simulink model "BEX6_USB_Torque_Control_HallSensor_BLDC_PMSM_2022b"  (R2022b)
settings: Solver=VariableStepAuto  StartTime=0.0  StopTime=inf  RelTol=1e-3
(part 1 of 2)
settings Model: Creator=SL_1  LastModifiedBy=SL_1
settings DebuggingCC: UnconnectedInputMsg=warning  UnconnectedOutputMsg=warning  UnconnectedLineMsg=warning
settings ModelReferenceCC: EnableRefExpFcnMdlSchedulingChecks=on
settings RTWCC: DLArmComputeVersion=19.05

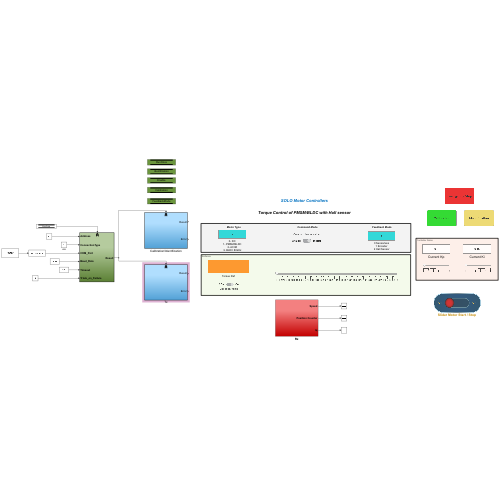
[thumbnail: Simulink's stored preview of the top-level diagram]
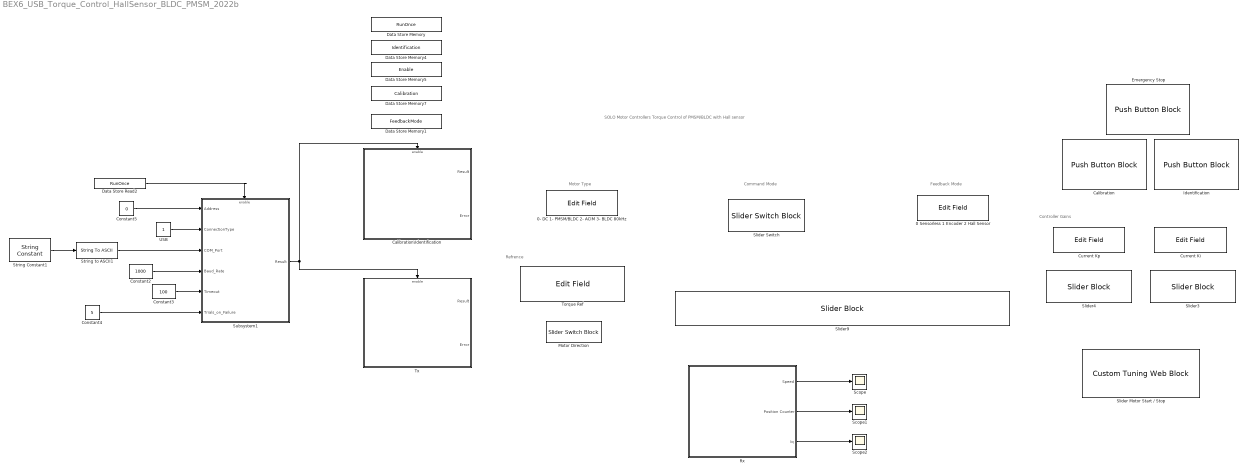
== system BEX6_USB_Torque_Control_HallSensor_BLDC_PMSM_2022b ==
  note: Command Mode
  note: Feedback Mode
  note: Refrence
  note: Controller Gains
  note: SOLO Motor Controllers
      |
      | Torque Control of PMSM/BLDC with Hall sensor
  note: Motor Type
  0 Sensorless 1 Encoder 2 Hall Sensor : EditField  LabelPosition=Hide  ShowInitialText=on  Alignment=Center
  "0- DC 1- PMSM/BLDC 2- ACIM 3- BLDC 80kHz " : EditField  LabelPosition=Hide  ShowInitialText=on  Alignment=Center
  Calibration : PushButtonBlock  ButtonText=Calibration  OffValue=0.000000
  Calibration\Identification : Subsystem
  Constant2 : Constant  Value=1000  OutDataTypeStr=uint32
  Constant3 : Constant  Value=100  OutDataTypeStr=double
  Constant4 : Constant  Value=5  OutDataTypeStr=int32
  Constant5 : Constant  Value=0  OutDataTypeStr=uint8
  Current Ki : EditField  LabelPosition=Hide  ShowInitialText=on  Alignment=Center
  Current Kp : EditField  LabelPosition=Hide  ShowInitialText=on  Alignment=Center
  Data Store Memory : DataStoreMemory  DataStoreName=RunOnce  ReadBeforeWriteMsg=warning  WriteAfterWriteMsg=warning  WriteAfterReadMsg=warning  InitialValue=1  ShowAdditionalParam=off  OutDataTypeStr=boolean
  Data Store Memory1 : DataStoreMemory  DataStoreName=FeedbackMode  ReadBeforeWriteMsg=warning  WriteAfterWriteMsg=warning  WriteAfterReadMsg=warning  ShowAdditionalParam=off
  Data Store Memory4 : DataStoreMemory  DataStoreName=Identification  ReadBeforeWriteMsg=warning  WriteAfterWriteMsg=warning  WriteAfterReadMsg=warning  ShowAdditionalParam=off
  Data Store Memory5 : DataStoreMemory  DataStoreName=Enable  ReadBeforeWriteMsg=warning  WriteAfterWriteMsg=warning  WriteAfterReadMsg=warning  ShowAdditionalParam=off
  Data Store Memory7 : DataStoreMemory  DataStoreName=Calibration  ReadBeforeWriteMsg=warning  WriteAfterWriteMsg=warning  WriteAfterReadMsg=warning  ShowAdditionalParam=off
  Data Store Read2 : DataStoreRead  DataStoreName=RunOnce  IndexOptions=Index vector (dialog)  Indices=1  OutputSizes=1
  Emergency Stop : PushButtonBlock  ButtonText=Emergency Stop  OnValue=0  OffValue=1.000000
  Identification : PushButtonBlock  ButtonText=Identification  OffValue=0.000000
  Motor Direction : SliderSwitchBlock  LabelPosition=Bottom
      settings: Values={{'CCw', 'Cw'}, [1 0]}
  Rx : Subsystem
  Scope : Scope
  Scope1 : Scope
  Scope2 : Scope
  Slider Motor Start / Stop : CustomTuningWebBlock  LabelPosition=Hide  ShowInitialText=on  Configuration="{\"type\":\"Switch\",\"settings\":{\"BindingType\":\"param\",\"backgroundColor\":[0,0,255,\"1\"],\"fixedAspectRatio\":\"on\",\"foregroundColor\":[234,234,234],\"showBackgroundColor\":false,\"variant\":\"slider\",\"version\":\"R2022b\"},\"components\":[{\"name\":\"CustomSwitchStateComponent\",\"settings\":{\"position\":[0,0,1,1],\"states\":[{\"HitRegion\":{\"position\":[0,0,0.5,1]},\"Image\":{\"position\":[0,0,1,1],\"size\":[1,1],\"src\":\"data:image/svg+xml;base64,PD94bWwgdmVyc2lvbj0iMS4wIiBlbmNvZGluZz0idXRmLTgiPz4NCjwhLS0gR2VuZXJhdG9yOiBBZG9iZSBJbGx1c3RyYXRvciAyNS4yLjEsIFNWRyBFeHBvcnQgUGx1Zy1JbiAuIFNWRyBWZXJzaW9uOiA2LjAwIEJ1aWxkIDApICAtLT4NCjxzdmcgdmVyc2lvbj0iMS4xIiB4bWxucz0iaHR0cDovL3d3dy53My5vcmcvMjAwMC9zdmciIHhtbG5zOnhsaW5rPSJodHRwOi8vd3d3LnczLm9yZy8xOTk5L3hsaW5rIiB4PSIwcHgiIHk9IjBweCINCgkgdmlld0JveD0iMCAwIDc2IDI5IiBzdHlsZT0iZW5hYmxlLWJhY2tncm91bmQ6bmV3 ...(+5404 chars)\",\"srcOrientation\":\"Right\"},\"Label\":{\"color\":[0.9294117647058824,0.6941176470588235,0.12549019607843137],\"icon\":{\"size\":[0,0],\"src\":[],\"srcOrientation\":\"Right\"},\"iconPlacement\":\"left\",\"opacity\":1,\"position\":[0.5,0.14],\"show\":true,\"text\":{\"content\":\"Off\",\"font\":\"Helvetica\",\"fontSize\":9}},\"Value\":0},{\"HitRegion\":{\"position\":[0,0.5,0.5,1]},\"Image\":{\"position\":[0,0,1,1],\"size\":[1,1],\"src\":\"data:image/svg+xml;base64,PD94bWwgdmVyc2lvbj0iMS4wIiBlbmNvZGluZz0idXRmLTgiPz4NCjwhLS0gR2VuZXJhdG9yOiBBZG9iZSBJbGx1c3RyYXRvciAyNS4yLjEsIFNWRyBFeHBvcnQgUGx1Zy1JbiAuIFNWRyBWZXJzaW9uOiA2LjAwIEJ1aWxkIDApICAtLT4NCjxzdmcgdmVyc2lvbj0iMS4xIiB4bWxucz0iaHR0cDovL3d3dy53My5vcmcvMjAwMC9zdmciIHhtbG5zOnhsaW5rPSJodHRwOi8vd3d3LnczLm9yZy8xOTk5L3hsaW5rIiB4PSIwcHgiIHk9IjBweCINCgkgdmlld0JveD0iMCAwIDc2IDI5IiBzdHlsZT0iZW5hYmxlLWJhY2tncm91bmQ6bmV3 ...(+5404 chars)\",\"srcOrientation\":\"Right\"},\"Label\":{\"color\":[0.9294117647058824,0.6941176470588235,0.12549019607843137],\"icon\":{\"size\":[0,0],\"src\":[],\"srcOrientation\":\"Right\"},\"iconPlacement\":\"left\",\"opacity\":1,\"position\":[0.5,0.86],\"show\":true,\"text\":{\"content\":\"On\",\"font\":\"Helvetica\",\"fontSize\":9}},\"Value\":1}]}},{\"name\":\"BackgroundImageComponent\",\"settings\":{\"image\":{\"size\":[0,0],\"src\":\"default\",\"srcOrientation\":[]},\"position\":[0,0,1,1],\"scaleMode\":\"0\"}},{\"name\":\"ForegroundImageComponent\",\"settings\":{\"image\":{\"size\":[0,0],\"src\":\"default\",\"srcOrientation\":[]},\"isForeground\":1,\"position\":[0,0,1,1],\"scaleMode\":\"0\"}}]}"
  Slider Switch : SliderSwitchBlock
      settings: Values={{'Analog', 'Digital'}, [0 1]}
  Slider3 : SliderBlock  LabelPosition=Hide  ScaleMax=5
  Slider4 : SliderBlock  LabelPosition=Hide  ScaleMax=5
  Slider9 : SliderBlock  LabelPosition=Hide  ScaleMax=3
  String Constant1 : StringConstant  String="\"COM5\""
  String to ASCII1 : StringToASCII  OutputVectorSize=5
  Subsystem1 : Subsystem
  Torque Ref : EditField  LabelPosition=Hide  ShowInitialText=on  Alignment=Center
  Tx : Subsystem
  USB : Constant  OutDataTypeStr=uint8
  wires:
  Rx/1(Speed) -> Scope/1
  Rx/2(Position Counter) -> Scope1/1
  Rx/3(Iq) -> Scope2/1
  Subsystem1/1(Result) -> Calibration\Identification/Enable, Tx/Enable
  Constant3/1 -> Subsystem1/5(Timeout)
  String to ASCII1/1 -> Subsystem1/3(COM_Port)
  Constant4/1 -> Subsystem1/6(Trials_on_Failure)
  Constant5/1 -> Subsystem1/1(Address)
  Constant2/1 -> Subsystem1/4(Baud_Rate)
  Data Store Read2/1 -> Subsystem1/Enable
  String Constant1/1 -> String to ASCII1/1
  USB/1 -> Subsystem1/2(ConnectionType)

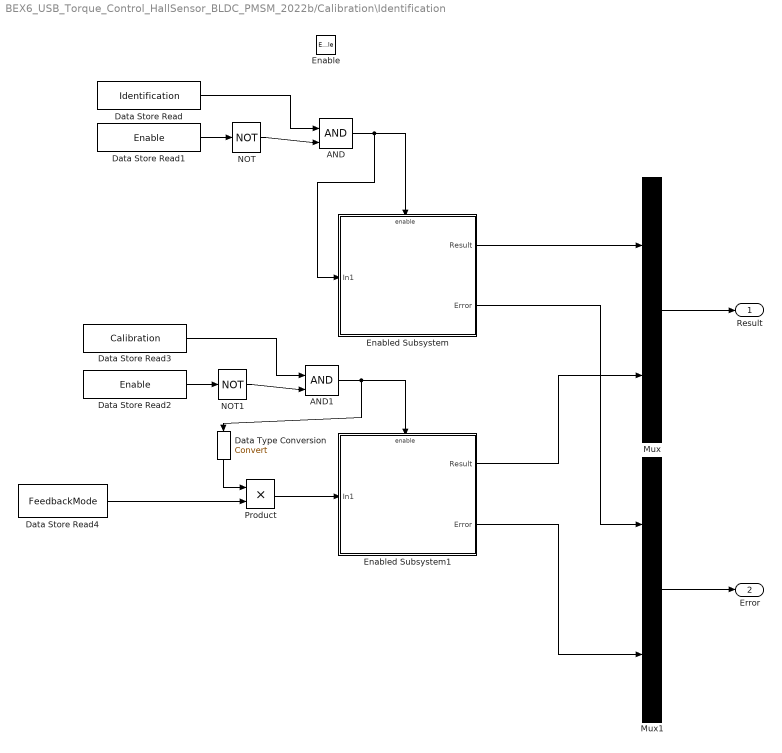
== system BEX6_USB_Torque_Control_HallSensor_BLDC_PMSM_2022b/Calibration\Identification ==
  Enable : EnablePort
  AND : Logic  IconShape=distinctive  AllPortsSameDT=off  OutDataTypeStr=boolean
  AND1 : Logic  IconShape=distinctive  AllPortsSameDT=off  OutDataTypeStr=boolean
  Data Store Read : DataStoreRead  DataStoreName=Identification  IndexOptions=Index vector (dialog)  Indices=1  OutputSizes=1
  Data Store Read1 : DataStoreRead  DataStoreName=Enable  IndexOptions=Index vector (dialog)  Indices=1  OutputSizes=1
  Data Store Read2 : DataStoreRead  DataStoreName=Enable  IndexOptions=Index vector (dialog)  Indices=1  OutputSizes=1
  Data Store Read3 : DataStoreRead  DataStoreName=Calibration  IndexOptions=Index vector (dialog)  Indices=1  OutputSizes=1
  Data Store Read4 : DataStoreRead  DataStoreName=FeedbackMode  IndexOptions=Index vector (dialog)  Indices=1  OutputSizes=1
  Data Type Conversion : DataTypeConversion  SaturateOnIntegerOverflow=off  RndMeth=Floor
  Enabled Subsystem : Subsystem  TreatAsAtomicUnit=on
  Enabled Subsystem1 : Subsystem  TreatAsAtomicUnit=on
  Mux : Mux  Inputs=2
  Mux1 : Mux  Inputs=2
  NOT : Logic  Operator=NOT  IconShape=distinctive  AllPortsSameDT=off  OutDataTypeStr=boolean
  NOT1 : Logic  Operator=NOT  IconShape=distinctive  AllPortsSameDT=off  OutDataTypeStr=boolean
  Product : Product
  Result : Outport
  Error : Outport  Port=2
  wires:
  Data Store Read1/1 -> NOT/1
  AND/1 -> Enabled Subsystem/1(In1), Enabled Subsystem/Enable
  NOT/1 -> AND/2
  Data Store Read/1 -> AND/1
  NOT1/1 -> AND1/2
  Data Store Read2/1 -> NOT1/1
  AND1/1 -> Data Type Conversion/1, Enabled Subsystem1/Enable
  Data Store Read3/1 -> AND1/1
  Enabled Subsystem1/2(Error) -> Mux1/2
  Enabled Subsystem1/1(Result) -> Mux/2
  Enabled Subsystem/1(Result) -> Mux/1
  Enabled Subsystem/2(Error) -> Mux1/1
  Mux1/1 -> Error/1
  Mux/1 -> Result/1
  Data Store Read4/1 -> Product/2
  Data Type Conversion/1 -> Product/1
  Product/1 -> Enabled Subsystem1/1(In1)

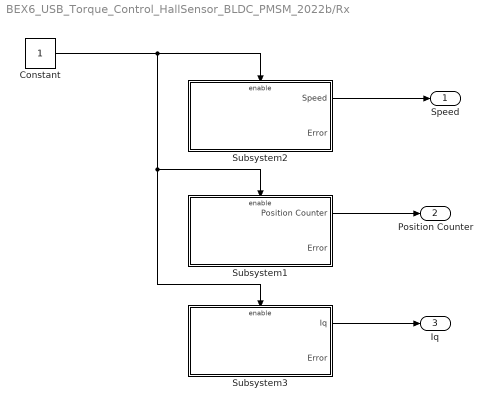
== system BEX6_USB_Torque_Control_HallSensor_BLDC_PMSM_2022b/Rx ==
  Constant : Constant  SampleTime=1e-3
  Subsystem1 : Subsystem
  Subsystem2 : Subsystem
  Subsystem3 : Subsystem
  Speed : Outport
  Position Counter : Outport  Port=2
  Iq : Outport  Port=3
  wires:
  Constant/1 -> Subsystem1/Enable, Subsystem3/Enable, Subsystem2/Enable
  Subsystem2/1(Speed) -> Speed/1
  Subsystem1/1(Position Counter) -> Position Counter/1
  Subsystem3/1(Iq) -> Iq/1

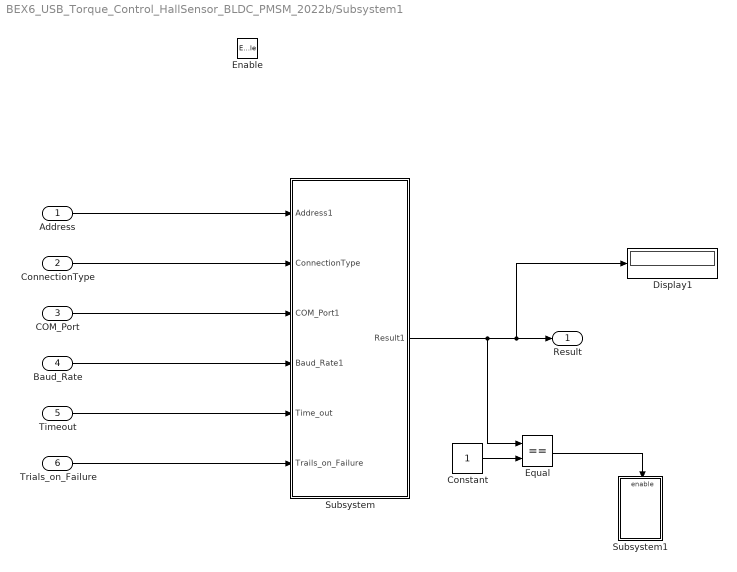
== system BEX6_USB_Torque_Control_HallSensor_BLDC_PMSM_2022b/Subsystem1 ==
  Address : Inport
  ConnectionType : Inport  Port=2
  COM_Port : Inport  Port=3
  Baud_Rate : Inport  Port=4
  Timeout : Inport  Port=5
  Trials_on_Failure : Inport  Port=6
  Enable : EnablePort
  Constant : Constant  OutDataTypeStr=Inherit: Inherit via back propagation
  Display1 : Display
  Equal : RelationalOperator  Operator===  OutDataTypeStr=boolean  RndMeth=Simplest  InputSameDT=off
  Subsystem : Subsystem
  Subsystem1 : Subsystem
  Result : Outport
  wires:
  Address/1 -> Subsystem/1(Address1)
  COM_Port/1 -> Subsystem/3(COM_Port1)
  Baud_Rate/1 -> Subsystem/4(Baud_Rate1)
  Timeout/1 -> Subsystem/5(Time_out)
  Trials_on_Failure/1 -> Subsystem/6(Trails_on_Failure)
  Equal/1 -> Subsystem1/Enable
  Subsystem/1(Result1) -> Display1/1, Result/1, Equal/1
  Constant/1 -> Equal/2
  ConnectionType/1 -> Subsystem/2(ConnectionType)

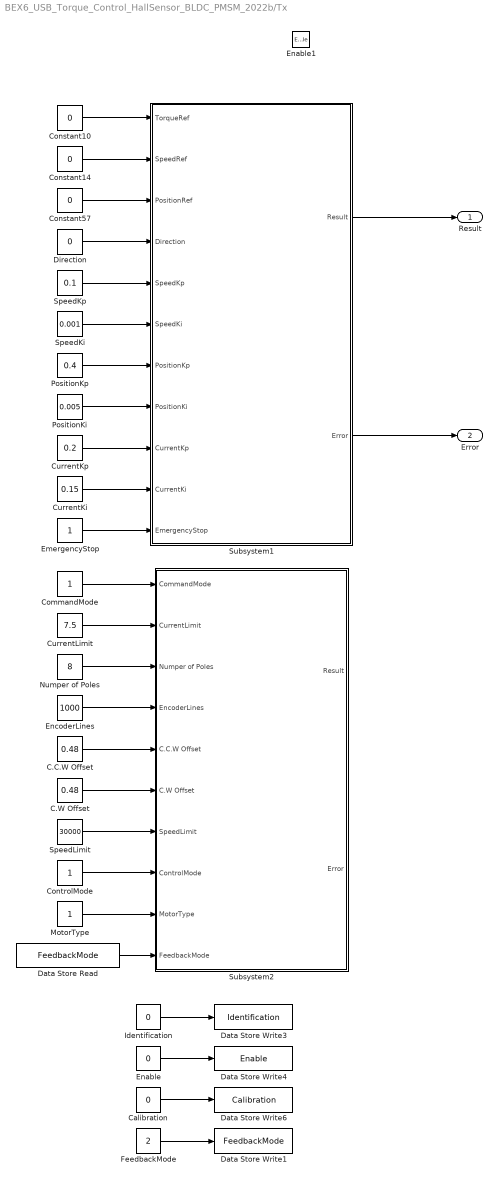
== system BEX6_USB_Torque_Control_HallSensor_BLDC_PMSM_2022b/Tx ==
  Enable1 : EnablePort
  C.C.W Offset : Constant  Value=0.48  OutDataTypeStr=Inherit: Inherit via back propagation
  C.W Offset : Constant  Value=0.48  OutDataTypeStr=Inherit: Inherit via back propagation
  Calibration : Constant  Value=0  OutDataTypeStr=Inherit: Inherit via back propagation
  CommandMode : Constant  OutDataTypeStr=Inherit: Inherit via back propagation
  Constant10 : Constant  Value=0  OutDataTypeStr=Inherit: Inherit via back propagation
  Constant14 : Constant  Value=0  OutDataTypeStr=Inherit: Inherit via back propagation
  Constant57 : Constant  Value=0  OutDataTypeStr=int32
  ControlMode : Constant  OutDataTypeStr=Inherit: Inherit via back propagation
  CurrentKi : Constant  Value=0.15  OutDataTypeStr=Inherit: Inherit via back propagation
  CurrentKp : Constant  Value=0.2  OutDataTypeStr=Inherit: Inherit via back propagation
  CurrentLimit : Constant  Value=7.5  OutDataTypeStr=Inherit: Inherit via back propagation
  Data Store Read : DataStoreRead  DataStoreName=FeedbackMode  IndexOptions=Index vector (dialog)  Indices=1  OutputSizes=1
  Data Store Write1 : DataStoreWrite  DataStoreName=FeedbackMode  IndexOptions=Index vector (dialog)  Indices=1  OutputSizes=1
  Data Store Write3 : DataStoreWrite  DataStoreName=Identification  IndexOptions=Index vector (dialog)  Indices=1  OutputSizes=1
  Data Store Write4 : DataStoreWrite  DataStoreName=Enable  IndexOptions=Index vector (dialog)  Indices=1  OutputSizes=1
  Data Store Write6 : DataStoreWrite  DataStoreName=Calibration  IndexOptions=Index vector (dialog)  Indices=1  OutputSizes=1
  Direction : Constant  Value=0  OutDataTypeStr=Inherit: Inherit via back propagation
  EmergencyStop : Constant  OutDataTypeStr=boolean
  Enable : Constant  Value=0  OutDataTypeStr=Inherit: Inherit via back propagation
  EncoderLines : Constant  Value=1000  OutDataTypeStr=Inherit: Inherit via back propagation
  FeedbackMode : Constant  Value=2  OutDataTypeStr=Inherit: Inherit via back propagation
  Identification : Constant  Value=0  OutDataTypeStr=Inherit: Inherit via back propagation
  MotorType : Constant  OutDataTypeStr=Inherit: Inherit via back propagation
  Numper of Poles : Constant  Value=8  OutDataTypeStr=Inherit: Inherit via back propagation
  PositionKi : Constant  Value=0.005  OutDataTypeStr=Inherit: Inherit via back propagation
  PositionKp : Constant  Value=0.4  OutDataTypeStr=Inherit: Inherit via back propagation
  SpeedKi : Constant  Value=0.001  OutDataTypeStr=Inherit: Inherit via back propagation
  SpeedKp : Constant  Value=0.1  OutDataTypeStr=Inherit: Inherit via back propagation
  SpeedLimit : Constant  Value=30000  OutDataTypeStr=Inherit: Inherit via back propagation
  Subsystem1 : Subsystem
  Subsystem2 : Subsystem
  Result : Outport
  Error : Outport  Port=2
  wires:
  Direction/1 -> Subsystem1/4(Direction)
  Constant10/1 -> Subsystem1/1(TorqueRef)
  Constant14/1 -> Subsystem1/2(SpeedRef)
  Constant57/1 -> Subsystem1/3(PositionRef)
  CurrentKi/1 -> Subsystem1/10(CurrentKi)
  CurrentKp/1 -> Subsystem1/9(CurrentKp)
  PositionKi/1 -> Subsystem1/8(PositionKi)
  PositionKp/1 -> Subsystem1/7(PositionKp)
  SpeedKi/1 -> Subsystem1/6(SpeedKi)
  SpeedKp/1 -> Subsystem1/5(SpeedKp)
  Identification/1 -> Data Store Write3/1
  Enable/1 -> Data Store Write4/1
  EmergencyStop/1 -> Subsystem1/11(EmergencyStop)
  Subsystem1/1(Result) -> Result/1
  Subsystem1/2(Error) -> Error/1
  C.C.W Offset/1 -> Subsystem2/5(C.C.W Offset)
  Numper of Poles/1 -> Subsystem2/3(Numper of Poles)
  SpeedLimit/1 -> Subsystem2/7(SpeedLimit)
  C.W Offset/1 -> Subsystem2/6(C.W Offset)
  CommandMode/1 -> Subsystem2/1(CommandMode)
  EncoderLines/1 -> Subsystem2/4(EncoderLines)
  CurrentLimit/1 -> Subsystem2/2(CurrentLimit)
  MotorType/1 -> Subsystem2/9(MotorType)
  FeedbackMode/1 -> Data Store Write1/1
  Data Store Read/1 -> Subsystem2/10(FeedbackMode)
  ControlMode/1 -> Subsystem2/8(ControlMode)
  Calibration/1 -> Data Store Write6/1

== system BEX6_USB_Torque_Control_HallSensor_BLDC_PMSM_2022b/Calibration\Identification/Enabled Subsystem ==
  In1 : Inport
  Enable : EnablePort
  Constant21 : Constant  Value=0  OutDataTypeStr=uint8
  MotorParameterIdentification : Subsystem
  Result : Outport
  Error : Outport  Port=2
  wires:
  In1/1 -> MotorParameterIdentification/2(Value)
  Constant21/1 -> MotorParameterIdentification/1(Address)
  MotorParameterIdentification/2(Error) -> Error/1
  MotorParameterIdentification/1(Result) -> Result/1

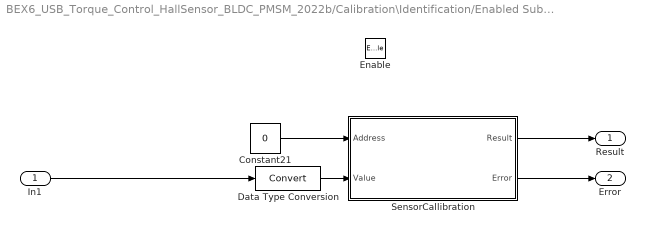
== system BEX6_USB_Torque_Control_HallSensor_BLDC_PMSM_2022b/Calibration\Identification/Enabled Subsystem1 ==
  In1 : Inport
  Enable : EnablePort
  Constant21 : Constant  Value=0  OutDataTypeStr=uint8
  Data Type Conversion : DataTypeConversion  SaturateOnIntegerOverflow=off  RndMeth=Floor
  SensorCallibration : Subsystem
  Result : Outport
  Error : Outport  Port=2
  wires:
  Constant21/1 -> SensorCallibration/1(Address)
  In1/1 -> Data Type Conversion/1
  Data Type Conversion/1 -> SensorCallibration/2(Value)
  SensorCallibration/2(Error) -> Error/1
  SensorCallibration/1(Result) -> Result/1

== system BEX6_USB_Torque_Control_HallSensor_BLDC_PMSM_2022b/Rx/Subsystem1 ==
  Enable : EnablePort
  Constant120 : Constant  Value=0  OutDataTypeStr=uint8
  GetPositionCountsFeedback : Subsystem
  Position Counter : Outport
  Error : Outport  Port=2
  wires:
  Constant120/1 -> GetPositionCountsFeedback/1(Address)
  GetPositionCountsFeedback/1(Result) -> Position Counter/1
  GetPositionCountsFeedback/2(Error) -> Error/1

== system BEX6_USB_Torque_Control_HallSensor_BLDC_PMSM_2022b/Rx/Subsystem2 ==
  Enable : EnablePort
  Constant120 : Constant  Value=0  OutDataTypeStr=uint8
  GetSpeedFeedback : Subsystem
  Speed : Outport
  Error : Outport  Port=2
  wires:
  GetSpeedFeedback/1(Result) -> Speed/1
  Constant120/1 -> GetSpeedFeedback/1(Address)
  GetSpeedFeedback/2(Error) -> Error/1

== system BEX6_USB_Torque_Control_HallSensor_BLDC_PMSM_2022b/Rx/Subsystem3 ==
  Enable : EnablePort
  Constant120 : Constant  Value=0  OutDataTypeStr=uint8
  GetQuadratureCurrentIqFeedback : Subsystem
  Iq : Outport
  Error : Outport  Port=2
  wires:
  GetQuadratureCurrentIqFeedback/2(Error) -> Error/1
  GetQuadratureCurrentIqFeedback/1(Result) -> Iq/1
  Constant120/1 -> GetQuadratureCurrentIqFeedback/1(Address)

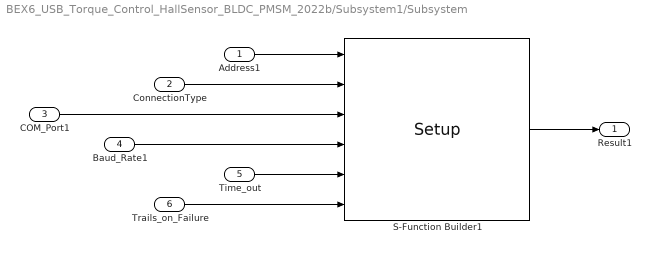
== system BEX6_USB_Torque_Control_HallSensor_BLDC_PMSM_2022b/Subsystem1/Subsystem ==
  Address1 : Inport
  ConnectionType : Inport  Port=2
  COM_Port1 : Inport  Port=3
  Baud_Rate1 : Inport  Port=4
  Time_out : Inport  Port=5
  Trails_on_Failure : Inport  Port=6
  S-Function Builder1 : S-Function  Priority=1  FunctionName=Setup  SFunctionModules=Setup_wrapper  SFunctionDeploymentMode=off  EnableBusSupport=off  mask(S-Function Builder){}
      mask help: Simulink:masks:SFunctionBuilder_MD
      mask init:
      | val = [[.9  0.75 0.75 1 1 .9 .9 1]',[1 1 0.75 0.75 .9 .9 1 .9]'];try , sys = get_param(gcb,'SfunBuilderFcnName');if isempty(sys), sys = get_param(gcb,'FunctionName'); end,catch, sys = get_param(gcb,'FunctionName'); end
      settings: CopyFcn=set_param(gcbh,'LinkStatus','none')  OpenFcn=sfunctionwizard(gcbh)
      mask Display:
      | plot(val(:,1),val(:,2))
      | disp(sys)
      | port_label('input',1,'Address')
      | port_label('input',2,'ConnectionType')
      | port_label('input',3,'COM_Port')
      | port_label('input',4,'Baud_Rate')
      | port_label('input',5,'Timeout')
      | port_label('input',6,'Trials_on_Failure')
      | port_label('output',1,'Result')
  Result1 : Outport
  wires:
  ConnectionType/1 -> S-Function Builder1/2
  Address1/1 -> S-Function Builder1/1
  S-Function Builder1/1 -> Result1/1
  Trails_on_Failure/1 -> S-Function Builder1/6
  COM_Port1/1 -> S-Function Builder1/3
  Time_out/1 -> S-Function Builder1/5
  Baud_Rate1/1 -> S-Function Builder1/4

== system BEX6_USB_Torque_Control_HallSensor_BLDC_PMSM_2022b/Subsystem1/Subsystem1 ==
  Enable : EnablePort
  Constant1 : Constant  Value=0  OutDataTypeStr=Inherit: Inherit via back propagation
  Data Store Write : DataStoreWrite  DataStoreName=RunOnce  IndexOptions=Index vector (dialog)  Indices=1  OutputSizes=1
  wires:
  Constant1/1 -> Data Store Write/1

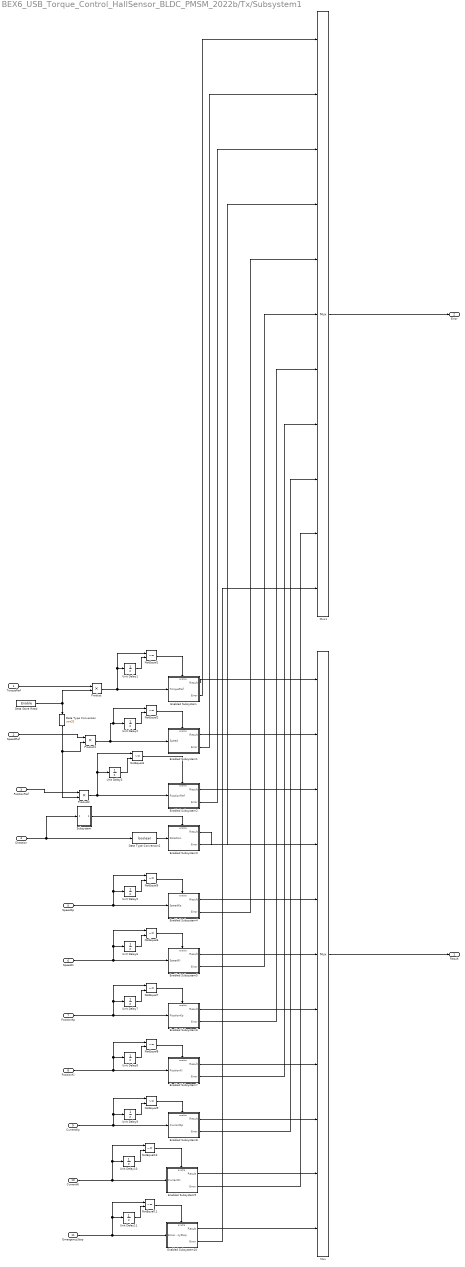
== system BEX6_USB_Torque_Control_HallSensor_BLDC_PMSM_2022b/Tx/Subsystem1 ==
  TorqueRef : Inport
  SpeedRef : Inport  Port=2
  PositionRef : Inport  Port=3
  Direction : Inport  Port=4
  SpeedKp : Inport  Port=5
  SpeedKi : Inport  Port=6
  PositionKp : Inport  Port=7
  PositionKi : Inport  Port=8
  CurrentKp : Inport  Port=9
  CurrentKi : Inport  Port=10
  EmergencyStop : Inport  Port=11
  Data Store Read : DataStoreRead  DataStoreName=Enable  IndexOptions=Index vector (dialog)  Indices=1  OutputSizes=1
  Data Type Conversion : DataTypeConversion  OutDataTypeStr=uint32  SaturateOnIntegerOverflow=off  RndMeth=Floor
  Data Type Conversion2 : DataTypeConversion  OutDataTypeStr=boolean  SaturateOnIntegerOverflow=off  RndMeth=Floor
  Enabled Subsystem : Subsystem  TreatAsAtomicUnit=on
  Enabled Subsystem1 : Subsystem  TreatAsAtomicUnit=on
  Enabled Subsystem10 : Subsystem  TreatAsAtomicUnit=on
  Enabled Subsystem2 : Subsystem  TreatAsAtomicUnit=on
  Enabled Subsystem3 : Subsystem  TreatAsAtomicUnit=on
  Enabled Subsystem4 : Subsystem  TreatAsAtomicUnit=on
  Enabled Subsystem5 : Subsystem  TreatAsAtomicUnit=on
  Enabled Subsystem6 : Subsystem  TreatAsAtomicUnit=on
  Enabled Subsystem7 : Subsystem  TreatAsAtomicUnit=on
  Enabled Subsystem8 : Subsystem  TreatAsAtomicUnit=on
  Enabled Subsystem9 : Subsystem  TreatAsAtomicUnit=on
  Mux : Mux  Inputs=11
  Mux1 : Mux  Inputs=11
  NotEqual{1..3,5..11} (10 alike) : RelationalOperator  Operator=~=  OutDataTypeStr=boolean  RndMeth=Simplest  InputSameDT=off
  Product : Product
  Product1 : Product  OutDataTypeStr=Inherit: Inherit via back propagation
  Product2 : Product  OutDataTypeStr=Inherit: Inherit via back propagation
  Subsystem : Subsystem
  Unit Delay{1..3,5..11} (10 alike) : UnitDelay  InitialCondition=2.1651  SampleTime=-1  HasFrameUpgradeWarning=on
  Result : Outport
  Error : Outport  Port=2
  wires:
  TorqueRef/1 -> Product/1
  Unit Delay1/1 -> NotEqual1/2
  NotEqual1/1 -> Enabled Subsystem/Enable
  Data Store Read/1 -> Product/2, Data Type Conversion/1
  Product/1 -> Enabled Subsystem/1(TorqueRef), NotEqual1/1, Unit Delay1/1
  NotEqual2/1 -> Enabled Subsystem1/Enable
  Unit Delay2/1 -> NotEqual2/2
  SpeedRef/1 -> Product1/1
  Product1/1 -> NotEqual2/1, Unit Delay2/1, Enabled Subsystem1/1(Speed)
  PositionRef/1 -> Product2/1
  Unit Delay3/1 -> NotEqual3/2
  NotEqual3/1 -> Enabled Subsystem2/Enable
  Direction/1 -> Data Type Conversion2/1, Subsystem/1(In1)
  NotEqual5/1 -> Enabled Subsystem4/Enable
  Unit Delay5/1 -> NotEqual5/2
  SpeedKp/1 -> Unit Delay5/1, NotEqual5/1, Enabled Subsystem4/1(SpeedKp)
  SpeedKi/1 -> NotEqual6/1, Unit Delay6/1, Enabled Subsystem5/1(SpeedKi)
  Unit Delay6/1 -> NotEqual6/2
  NotEqual6/1 -> Enabled Subsystem5/Enable
  NotEqual7/1 -> Enabled Subsystem6/Enable
  Unit Delay7/1 -> NotEqual7/2
  PositionKp/1 -> Unit Delay7/1, NotEqual7/1, Enabled Subsystem6/1(PositionKp)
  PositionKi/1 -> NotEqual8/1, Unit Delay8/1, Enabled Subsystem7/1(PositionKi)
  Unit Delay8/1 -> NotEqual8/2
  NotEqual8/1 -> Enabled Subsystem7/Enable
  NotEqual9/1 -> Enabled Subsystem8/Enable
  Unit Delay9/1 -> NotEqual9/2
  CurrentKp/1 -> Unit Delay9/1, NotEqual9/1, Enabled Subsystem8/1(CurrentKp)
  CurrentKi/1 -> NotEqual10/1, Unit Delay10/1, Enabled Subsystem9/1(CurrentKi)
  Unit Delay10/1 -> NotEqual10/2
  NotEqual10/1 -> Enabled Subsystem9/Enable
  NotEqual11/1 -> Enabled Subsystem10/Enable
  Unit Delay11/1 -> NotEqual11/2
  EmergencyStop/1 -> Unit Delay11/1, NotEqual11/1, Enabled Subsystem10/1(EmergencyStop)
  Product2/1 -> NotEqual3/1, Unit Delay3/1, Enabled Subsystem2/1(PositionRef)
  Data Type Conversion2/1 -> Enabled Subsystem3/1(Direction)
  Enabled Subsystem/1(Result) -> Mux/1
  Enabled Subsystem10/1(Result) -> Mux/11
  Enabled Subsystem9/1(Result) -> Mux/10
  Enabled Subsystem8/1(Result) -> Mux/9
  Enabled Subsystem7/1(Result) -> Mux/8
  Enabled Subsystem6/1(Result) -> Mux/7
  Enabled Subsystem5/1(Result) -> Mux/6
  Enabled Subsystem4/1(Result) -> Mux/5
  Enabled Subsystem3/1(Result) -> Mux/4
  Enabled Subsystem2/1(Result) -> Mux/3
  Enabled Subsystem1/1(Result) -> Mux/2
  Mux/1 -> Result/1
  Enabled Subsystem/2(Error) -> Mux1/1
  Enabled Subsystem1/2(Error) -> Mux1/2
  Enabled Subsystem2/2(Error) -> Mux1/3
  Enabled Subsystem3/2(Error) -> Mux1/4
  Enabled Subsystem4/2(Error) -> Mux1/5
  Enabled Subsystem5/2(Error) -> Mux1/6
  Enabled Subsystem6/2(Error) -> Mux1/7
  Enabled Subsystem7/2(Error) -> Mux1/8
  Enabled Subsystem8/2(Error) -> Mux1/9
  Enabled Subsystem9/2(Error) -> Mux1/10
  Enabled Subsystem10/2(Error) -> Mux1/11
  Mux1/1 -> Error/1
  Data Type Conversion/1 -> Product2/2, Product1/2
  Subsystem/1(Out1) -> Enabled Subsystem3/Enable

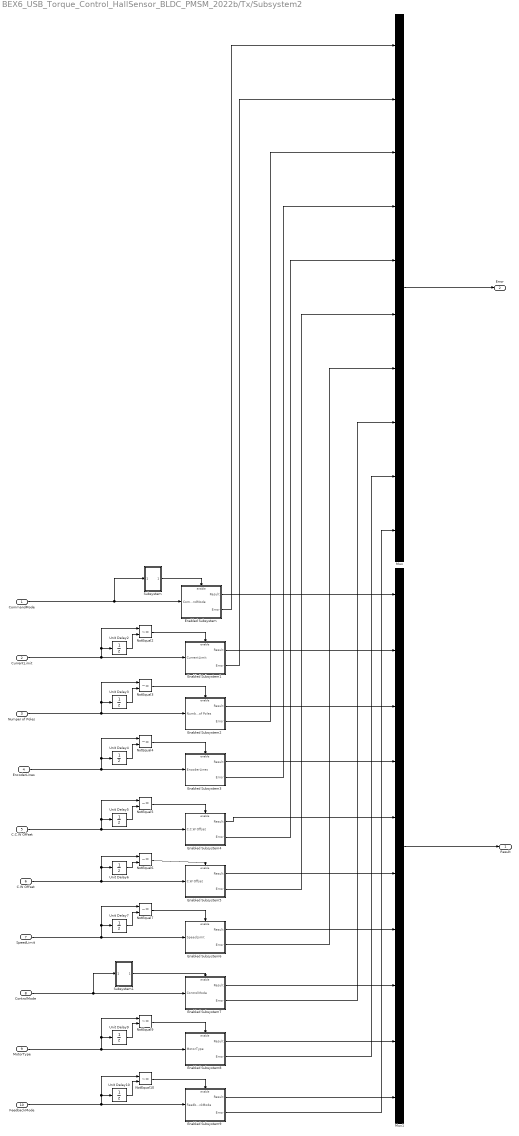
== system BEX6_USB_Torque_Control_HallSensor_BLDC_PMSM_2022b/Tx/Subsystem2 ==
  CommandMode : Inport
  CurrentLimit : Inport  Port=2
  Numper of Poles : Inport  Port=3
  EncoderLines : Inport  Port=4
  C.C.W Offset : Inport  Port=5
  C.W Offset : Inport  Port=6
  SpeedLimit : Inport  Port=7
  ControlMode : Inport  Port=8
  MotorType : Inport  Port=9
  FeedbackMode : Inport  Port=10
  Enabled Subsystem : Subsystem  TreatAsAtomicUnit=on
  Enabled Subsystem1 : Subsystem  TreatAsAtomicUnit=on
  Enabled Subsystem2 : Subsystem  TreatAsAtomicUnit=on
  Enabled Subsystem3 : Subsystem  TreatAsAtomicUnit=on
  Enabled Subsystem4 : Subsystem  TreatAsAtomicUnit=on
  Enabled Subsystem5 : Subsystem  TreatAsAtomicUnit=on
  Enabled Subsystem6 : Subsystem  TreatAsAtomicUnit=on
  Enabled Subsystem7 : Subsystem  TreatAsAtomicUnit=on
  Enabled Subsystem8 : Subsystem  TreatAsAtomicUnit=on
  Enabled Subsystem9 : Subsystem  TreatAsAtomicUnit=on
  Mux : Mux  Inputs=10
  Mux1 : Mux  Inputs=10
  NotEqual{2..7,9..10} (8 alike) : RelationalOperator  Operator=~=  OutDataTypeStr=boolean  RndMeth=Simplest  InputSameDT=off
  Subsystem : Subsystem
  Subsystem1 : Subsystem
  Unit Delay{2..7,9..10} (8 alike) : UnitDelay  InitialCondition=2.1651  SampleTime=-1  HasFrameUpgradeWarning=on
  Result : Outport
  Error : Outport  Port=2
  wires:
  NotEqual2/1 -> Enabled Subsystem1/Enable
  CurrentLimit/1 -> NotEqual2/1, Unit Delay2/1, Enabled Subsystem1/1(CurrentLimit)
  Unit Delay2/1 -> NotEqual2/2
  Unit Delay3/1 -> NotEqual3/2
  Numper of Poles/1 -> Enabled Subsystem2/1(Number of Poles), Unit Delay3/1, NotEqual3/1
  NotEqual3/1 -> Enabled Subsystem2/Enable
  NotEqual4/1 -> Enabled Subsystem3/Enable
  EncoderLines/1 -> NotEqual4/1, Unit Delay4/1, Enabled Subsystem3/1(EncoderLines)
  Unit Delay4/1 -> NotEqual4/2
  Unit Delay5/1 -> NotEqual5/2
  C.C.W Offset/1 -> Enabled Subsystem4/1(C.C.W Offset), Unit Delay5/1, NotEqual5/1
  NotEqual5/1 -> Enabled Subsystem4/Enable
  NotEqual6/1 -> Enabled Subsystem5/Enable
  C.W Offset/1 -> NotEqual6/1, Unit Delay6/1, Enabled Subsystem5/1(C.W Offset)
  Unit Delay6/1 -> NotEqual6/2
  Unit Delay7/1 -> NotEqual7/2
  SpeedLimit/1 -> Enabled Subsystem6/1(SpeedLimit), Unit Delay7/1, NotEqual7/1
  NotEqual7/1 -> Enabled Subsystem6/Enable
  ControlMode/1 -> Subsystem1/1(In1), Enabled Subsystem7/1(ControlMode)
  Unit Delay9/1 -> NotEqual9/2
  MotorType/1 -> Unit Delay9/1, NotEqual9/1, Enabled Subsystem8/1(MotorType)
  NotEqual9/1 -> Enabled Subsystem8/Enable
  NotEqual10/1 -> Enabled Subsystem9/Enable
  FeedbackMode/1 -> NotEqual10/1, Unit Delay10/1, Enabled Subsystem9/1(FeedbackMode)
  Unit Delay10/1 -> NotEqual10/2
  CommandMode/1 -> Subsystem/1(In1), Enabled Subsystem/1(CommandMode)
  Enabled Subsystem9/2(Error) -> Mux/10
  Enabled Subsystem8/2(Error) -> Mux/9
  Enabled Subsystem7/2(Error) -> Mux/8
  Enabled Subsystem6/2(Error) -> Mux/7
  Enabled Subsystem5/2(Error) -> Mux/6
  Enabled Subsystem4/2(Error) -> Mux/5
  Enabled Subsystem3/2(Error) -> Mux/4
  Enabled Subsystem2/2(Error) -> Mux/3
  Enabled Subsystem1/2(Error) -> Mux/2
  Enabled Subsystem/2(Error) -> Mux/1
  Enabled Subsystem/1(Result) -> Mux1/1
  Enabled Subsystem1/1(Result) -> Mux1/2
  Enabled Subsystem2/1(Result) -> Mux1/3
  Enabled Subsystem3/1(Result) -> Mux1/4
  Enabled Subsystem5/1(Result) -> Mux1/6
  Enabled Subsystem7/1(Result) -> Mux1/8
  Enabled Subsystem6/1(Result) -> Mux1/7
  Enabled Subsystem8/1(Result) -> Mux1/9
  Enabled Subsystem9/1(Result) -> Mux1/10
  Enabled Subsystem4/1(Result) -> Mux1/5
  Mux1/1 -> Result/1
  Mux/1 -> Error/1
  Subsystem/1(Out2) -> Enabled Subsystem/Enable
  Subsystem1/1(Out1) -> Enabled Subsystem7/Enable

== system BEX6_USB_Torque_Control_HallSensor_BLDC_PMSM_2022b/Calibration\Identification/Enabled Subsystem/MotorParameterIdentification ==
  Address : Inport
  Value : Inport  Port=2
  Display20 : Display
      settings: Format=decimal (Stored Integer)
  Display21 : Display
      settings: Format=decimal (Stored Integer)
  S-Function Builder10 : S-Function  Priority=2  FunctionName=MotorParametersIdentification  SFunctionModules=MotorParametersIdentification_wrapper  SFunctionDeploymentMode=off  EnableBusSupport=off  mask(S-Function Builder){}
      mask help: Simulink:masks:SFunctionBuilder_MD
      mask init: same as BEX6_USB_Torque_Control_HallSensor_BLDC_PMSM_2022b/Subsystem1/Subsystem/S-Function Builder1
      settings: CopyFcn=set_param(gcbh,'LinkStatus','none')  OpenFcn=sfunctionwizard(gcbh)
      mask Display:
      | plot(val(:,1),val(:,2))
      | disp(sys)
      | port_label('input',1,'Address')
      | port_label('input',2,'Value')
      | port_label('output',1,'Result')
      | port_label('output',2,'Error')
  Result : Outport
  Error : Outport  Port=2
  wires:
  S-Function Builder10/2 -> Error/1, Display21/1
  S-Function Builder10/1 -> Result/1, Display20/1
  Value/1 -> S-Function Builder10/2
  Address/1 -> S-Function Builder10/1

== system BEX6_USB_Torque_Control_HallSensor_BLDC_PMSM_2022b/Calibration\Identification/Enabled Subsystem1/SensorCallibration ==
  Address : Inport
  Value : Inport  Port=2
  S-Function Builder41 : S-Function  Priority=2  FunctionName=SensorCalibration  SFunctionModules=SensorCalibration_wrapper  SFunctionDeploymentMode=off  EnableBusSupport=off  mask(S-Function Builder){}
      mask help: Simulink:masks:SFunctionBuilder_MD
      mask init: same as BEX6_USB_Torque_Control_HallSensor_BLDC_PMSM_2022b/Subsystem1/Subsystem/S-Function Builder1
      settings: CopyFcn=set_param(gcbh,'LinkStatus','none')  OpenFcn=sfunctionwizard(gcbh)
      mask Display:
      | plot(val(:,1),val(:,2))
      | disp(sys)
      | port_label('input',1,'Address')
      | port_label('input',2,'Value')
      | port_label('output',1,'Result')
      | port_label('output',2,'Error')
  Result : Outport
  Error : Outport  Port=2
  wires:
  Value/1 -> S-Function Builder41/2
  S-Function Builder41/1 -> Result/1
  Address/1 -> S-Function Builder41/1
  S-Function Builder41/2 -> Error/1

== system BEX6_USB_Torque_Control_HallSensor_BLDC_PMSM_2022b/Rx/Subsystem1/GetPositionCountsFeedback ==
  Address : Inport
  S-Function Builder73 : S-Function  Priority=3  FunctionName=GetPositionCountsFeedback  SFunctionModules=GetPositionCountsFeedback_wrapper  SFunctionDeploymentMode=off  EnableBusSupport=off  mask(S-Function Builder){}
      mask help: Simulink:masks:SFunctionBuilder_MD
      mask init: same as BEX6_USB_Torque_Control_HallSensor_BLDC_PMSM_2022b/Subsystem1/Subsystem/S-Function Builder1
      settings: CopyFcn=set_param(gcbh,'LinkStatus','none')  OpenFcn=sfunctionwizard(gcbh)
      mask Display: plot(val(:,1),val(:,2)),disp(sys),port_label('input',1,'Address'),port_label('output',1,'Result'),port_label('output',2,'Error')
  Result : Outport
  Error : Outport  Port=2
  wires:
  Address/1 -> S-Function Builder73/1
  S-Function Builder73/2 -> Error/1
  S-Function Builder73/1 -> Result/1

== system BEX6_USB_Torque_Control_HallSensor_BLDC_PMSM_2022b/Rx/Subsystem2/GetSpeedFeedback ==
  Address : Inport
  S-Function Builder66 : S-Function  Priority=3  FunctionName=GetSpeedFeedback  SFunctionModules=GetSpeedFeedback_wrapper  SFunctionDeploymentMode=off  EnableBusSupport=off  mask(S-Function Builder){}
      mask help: Simulink:masks:SFunctionBuilder_MD
      mask init: same as BEX6_USB_Torque_Control_HallSensor_BLDC_PMSM_2022b/Subsystem1/Subsystem/S-Function Builder1
      settings: CopyFcn=set_param(gcbh,'LinkStatus','none')  OpenFcn=sfunctionwizard(gcbh)
      mask Display: plot(val(:,1),val(:,2)),disp(sys),port_label('input',1,'Address'),port_label('output',1,'Result'),port_label('output',2,'Error')
  Result : Outport
  Error : Outport  Port=2
  wires:
  Address/1 -> S-Function Builder66/1
  S-Function Builder66/1 -> Result/1
  S-Function Builder66/2 -> Error/1

== system BEX6_USB_Torque_Control_HallSensor_BLDC_PMSM_2022b/Rx/Subsystem3/GetQuadratureCurrentIqFeedback ==
  Address : Inport
  S-Function Builder57 : S-Function  Priority=3  FunctionName=GetQuadratureCurrentIqFeedback  SFunctionModules=GetQuadratureCurrentIqFeedback_wrapper  SFunctionDeploymentMode=off  EnableBusSupport=off  mask(S-Function Builder){}
      mask help: Simulink:masks:SFunctionBuilder_MD
      mask init: same as BEX6_USB_Torque_Control_HallSensor_BLDC_PMSM_2022b/Subsystem1/Subsystem/S-Function Builder1
      settings: CopyFcn=set_param(gcbh,'LinkStatus','none')  OpenFcn=sfunctionwizard(gcbh)
      mask Display: plot(val(:,1),val(:,2)),disp(sys),port_label('input',1,'Address'),port_label('output',1,'Result'),port_label('output',2,'Error')
  Result : Outport
  Error : Outport  Port=2
  wires:
  S-Function Builder57/2 -> Error/1
  Address/1 -> S-Function Builder57/1
  S-Function Builder57/1 -> Result/1

== system BEX6_USB_Torque_Control_HallSensor_BLDC_PMSM_2022b/Tx/Subsystem1/Enabled Subsystem ==
  TorqueRef : Inport
  Enable : EnablePort
  Constant : Constant  Value=0  OutDataTypeStr=Inherit: Inherit via back propagation
  SetTorqueReferenceIq : Subsystem
  Result : Outport
  Error : Outport  Port=2
  wires:
  Constant/1 -> SetTorqueReferenceIq/1(Address)
  TorqueRef/1 -> SetTorqueReferenceIq/2(Value)
  SetTorqueReferenceIq/1(Result) -> Result/1
  SetTorqueReferenceIq/2(Error) -> Error/1

== system BEX6_USB_Torque_Control_HallSensor_BLDC_PMSM_2022b/Tx/Subsystem1/Enabled Subsystem1 ==
  Speed : Inport
  Enable : EnablePort
  Constant : Constant  Value=0  OutDataTypeStr=Inherit: Inherit via back propagation
  SpeedRef : Subsystem
  Result : Outport
  Error : Outport  Port=2
  wires:
  Constant/1 -> SpeedRef/1(Address)
  Speed/1 -> SpeedRef/2(Value)
  SpeedRef/2(Error) -> Error/1
  SpeedRef/1(Result) -> Result/1

== system BEX6_USB_Torque_Control_HallSensor_BLDC_PMSM_2022b/Tx/Subsystem1/Enabled Subsystem10 ==
  EmergencyStop : Inport
  Enable : EnablePort
  Data Type Conversion : DataTypeConversion  SaturateOnIntegerOverflow=off  RndMeth=Floor
  EmergencyStop1 : Subsystem
  Result : Outport
  Error : Outport  Port=2
  wires:
  EmergencyStop/1 -> Data Type Conversion/1
  EmergencyStop1/2(Error) -> Error/1
  EmergencyStop1/1(Result) -> Result/1
  Data Type Conversion/1 -> EmergencyStop1/1(Address)

== system BEX6_USB_Torque_Control_HallSensor_BLDC_PMSM_2022b/Tx/Subsystem1/Enabled Subsystem2 ==
  PositionRef : Inport
  Enable : EnablePort
  Constant : Constant  Value=0  OutDataTypeStr=Inherit: Inherit via back propagation
  SetPositionRef : Subsystem
  Result : Outport
  Error : Outport  Port=2
  wires:
  PositionRef/1 -> SetPositionRef/2(Value)
  Constant/1 -> SetPositionRef/1(Address)
  SetPositionRef/2(Error) -> Error/1
  SetPositionRef/1(Result) -> Result/1

== system BEX6_USB_Torque_Control_HallSensor_BLDC_PMSM_2022b/Tx/Subsystem1/Enabled Subsystem3 ==
  Direction : Inport
  Enable : EnablePort
  Constant : Constant  Value=0  OutDataTypeStr=Inherit: Inherit via back propagation
  SetMotorDirection : Subsystem
  Result : Outport
  Error : Outport  Port=2
  wires:
  Constant/1 -> SetMotorDirection/1(Address)
  Direction/1 -> SetMotorDirection/2(Value)
  SetMotorDirection/2(Error) -> Error/1
  SetMotorDirection/1(Result) -> Result/1

== system BEX6_USB_Torque_Control_HallSensor_BLDC_PMSM_2022b/Tx/Subsystem1/Enabled Subsystem4 ==
  SpeedKp : Inport
  Enable : EnablePort
  Constant26 : Constant  Value=0  OutDataTypeStr=uint8
  SetSpeed Kp : Subsystem
  Result : Outport
  Error : Outport  Port=2
  wires:
  SetSpeed Kp/2(Error) -> Error/1
  SetSpeed Kp/1(Result) -> Result/1
  Constant26/1 -> SetSpeed Kp/1(Address)
  SpeedKp/1 -> SetSpeed Kp/2(Value)

== system BEX6_USB_Torque_Control_HallSensor_BLDC_PMSM_2022b/Tx/Subsystem1/Enabled Subsystem5 ==
  SpeedKi : Inport
  Enable : EnablePort
  Constant28 : Constant  Value=0  OutDataTypeStr=uint8
  SetSpeed Ki : Subsystem
  Result : Outport
  Error : Outport  Port=2
  wires:
  Constant28/1 -> SetSpeed Ki/1(Address)
  SpeedKi/1 -> SetSpeed Ki/2(Value)
  SetSpeed Ki/2(Error) -> Error/1
  SetSpeed Ki/1(Result) -> Result/1

== system BEX6_USB_Torque_Control_HallSensor_BLDC_PMSM_2022b/Tx/Subsystem1/Enabled Subsystem6 ==
  PositionKp : Inport
  Enable : EnablePort
  Constant60 : Constant  Value=0  OutDataTypeStr=uint8
  SetPositionControllerKp : Subsystem
  Result : Outport
  Error : Outport  Port=2
  wires:
  PositionKp/1 -> SetPositionControllerKp/2(Value)
  SetPositionControllerKp/2(Error) -> Error/1
  SetPositionControllerKp/1(Result) -> Result/1
  Constant60/1 -> SetPositionControllerKp/1(Address)

== system BEX6_USB_Torque_Control_HallSensor_BLDC_PMSM_2022b/Tx/Subsystem1/Enabled Subsystem7 ==
  PositionKi : Inport
  Enable : EnablePort
  Constant62 : Constant  Value=0  OutDataTypeStr=uint8
  SetPositionControllerKi : Subsystem
  Result : Outport
  Error : Outport  Port=2
  wires:
  PositionKi/1 -> SetPositionControllerKi/2(Value)
  SetPositionControllerKi/2(Error) -> Error/1
  SetPositionControllerKi/1(Result) -> Result/1
  Constant62/1 -> SetPositionControllerKi/1(Address)

== system BEX6_USB_Torque_Control_HallSensor_BLDC_PMSM_2022b/Tx/Subsystem1/Enabled Subsystem8 ==
  CurrentKp : Inport
  Enable : EnablePort
  Constant50 : Constant  Value=0  OutDataTypeStr=uint8
  SetCurrentControlKp : Subsystem
  Result : Outport
  Error : Outport  Port=2
  wires:
  CurrentKp/1 -> SetCurrentControlKp/2(Value)
  SetCurrentControlKp/2(Error) -> Error/1
  SetCurrentControlKp/1(Result) -> Result/1
  Constant50/1 -> SetCurrentControlKp/1(Address)

== system BEX6_USB_Torque_Control_HallSensor_BLDC_PMSM_2022b/Tx/Subsystem1/Enabled Subsystem9 ==
  CurrentKi : Inport
  Enable : EnablePort
  Constant52 : Constant  Value=0  OutDataTypeStr=uint8
  SetCurrentControlKi : Subsystem
  Result : Outport
  Error : Outport  Port=2
  wires:
  CurrentKi/1 -> SetCurrentControlKi/2(Value)
  SetCurrentControlKi/2(Error) -> Error/1
  SetCurrentControlKi/1(Result) -> Result/1
  Constant52/1 -> SetCurrentControlKi/1(Address)

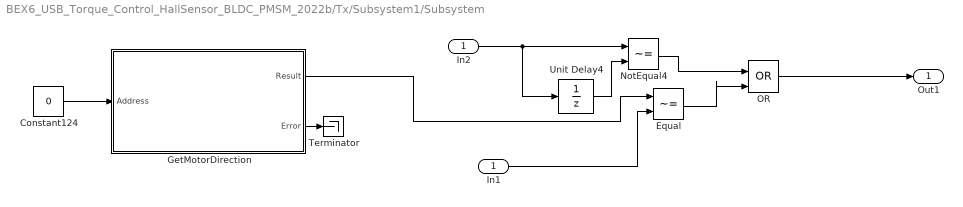
== system BEX6_USB_Torque_Control_HallSensor_BLDC_PMSM_2022b/Tx/Subsystem1/Subsystem ==
  In1 : Inport
  Constant124 : Constant  Value=0  OutDataTypeStr=uint8
  Equal : RelationalOperator  Operator=~=  OutDataTypeStr=boolean  RndMeth=Simplest  InputSameDT=off
  GetMotorDirection : Subsystem
  In2 : InportShadow
  NotEqual4 : RelationalOperator  Operator=~=  OutDataTypeStr=boolean  RndMeth=Simplest  InputSameDT=off
  OR : Logic  Operator=OR  IconShape=distinctive  AllPortsSameDT=off  OutDataTypeStr=boolean
  Terminator : Terminator
  Unit Delay4 : UnitDelay  InitialCondition=2.1651  SampleTime=-1  HasFrameUpgradeWarning=on
  Out1 : Outport
  wires:
  In2/1 -> Unit Delay4/1, NotEqual4/1
  NotEqual4/1 -> OR/1
  Equal/1 -> OR/2
  Unit Delay4/1 -> NotEqual4/2
  Constant124/1 -> GetMotorDirection/1(Address)
  GetMotorDirection/1(Result) -> Equal/1
  In1/1 -> Equal/2
  OR/1 -> Out1/1
  GetMotorDirection/2(Error) -> Terminator/1

== system BEX6_USB_Torque_Control_HallSensor_BLDC_PMSM_2022b/Tx/Subsystem2/Enabled Subsystem ==
  CommandMode : Inport
  Enable : EnablePort
  Constant6 : Constant  Value=0  OutDataTypeStr=Inherit: Inherit via back propagation
  SetCommandMode : Subsystem
  Result : Outport
  Error : Outport  Port=2
  wires:
  Constant6/1 -> SetCommandMode/1(Address)
  CommandMode/1 -> SetCommandMode/2(Value)
  SetCommandMode/1(Result) -> Result/1
  SetCommandMode/2(Error) -> Error/1

== system BEX6_USB_Torque_Control_HallSensor_BLDC_PMSM_2022b/Tx/Subsystem2/Enabled Subsystem1 ==
  CurrentLimit : Inport
  Enable : EnablePort
  Constant6 : Constant  Value=0  OutDataTypeStr=uint8
  SetCurrentLimit : Subsystem
  Result : Outport
  Error : Outport  Port=2
  wires:
  Constant6/1 -> SetCurrentLimit/1(Address)
  CurrentLimit/1 -> SetCurrentLimit/2(Value)
  SetCurrentLimit/2(Error) -> Error/1
  SetCurrentLimit/1(Result) -> Result/1

== system BEX6_USB_Torque_Control_HallSensor_BLDC_PMSM_2022b/Tx/Subsystem2/Enabled Subsystem2 ==
  Number of Poles : Inport
  Enable : EnablePort
  Constant6 : Constant  Value=0  OutDataTypeStr=uint8
  SetMotorPoleCounts : Subsystem
  Result : Outport
  Error : Outport  Port=2
  wires:
  Number of Poles/1 -> SetMotorPoleCounts/2(Value)
  Constant6/1 -> SetMotorPoleCounts/1(Address)
  SetMotorPoleCounts/2(Error) -> Error/1
  SetMotorPoleCounts/1(Result) -> Result/1

== system BEX6_USB_Torque_Control_HallSensor_BLDC_PMSM_2022b/Tx/Subsystem2/Enabled Subsystem3 ==
  EncoderLines : Inport
  Enable : EnablePort
  Constant6 : Constant  Value=0  OutDataTypeStr=uint8
  SetEncoderLines : Subsystem
  Result : Outport
  Error : Outport  Port=2
  wires:
  Constant6/1 -> SetEncoderLines/1(Address)
  EncoderLines/1 -> SetEncoderLines/2(Value)
  SetEncoderLines/2(Error) -> Error/1
  SetEncoderLines/1(Result) -> Result/1
